simulink model "tutorial_switched_nets"  (R2020a)
settings: Solver=FixedStepAuto  StartTime=0.0  StopTime=options.T_train  FixedStep=options.dt  MaxStep=.2  RelTol=1e-3
model workspace (MAT data in the model file):
  PID_TRESH = 0.3
undefined symbols (not defined in the file or in its folder): DiscIntNeverNeededParam, options
libraries: neural x72, simulink x2
(part 2 of 3)

== system tutorial_switched_nets/NN/Layer 2/Delays 1 ==
  "p{2}" : Inport  PortDimensions=20
      mask Display: e = 0.06;c1 = [120 230 180]/255;c2 = ([120 230 180]+0)/(256+128);c3 = ([120 230 180]+128)/(256+128);patch([0 1 1 0],[0 0 1 1],c1);patch([0 1 1 1-e 1-e 0+e],[0 0 1 1-e 0+e 0+e],c2);patch([0 0 1 1-e 0+e 0+e],[0 1 1 1-e 1-e 0+e],c3);plot([0 1 1 0 0],[0 0 1 1 0]);
  mux : Mux  Inputs=1
      mask Display: e = 0.06;c1 = [120 150 230]/255;c2 = ([120 150 230]+0)/383;c3 = ([120 150 230]+128)/383;patch([0 1 1 0],[0 0 1 1],c1);patch([0 1 1 1-e 1-e 0+e],[0 0 1 1-e 0+e 0+e],c2);patch([0 0 1 1-e 0+e 0+e],[0 1 1 1-e 1-e 0+e],c3);plot([0 1 1 0 0],[0 0 1 1 0]);disp('Mux')
  "pd{2,1}" : Outport
      mask Display: e = 0.06;c1 = [120 230 180]/255;c2 = ([120 230 180]+0)/(256+128);c3 = ([120 230 180]+128)/(256+128);patch([0 1 1 0],[0 0 1 1],c1);patch([0 1 1 1-e 1-e 0+e],[0 0 1 1-e 0+e 0+e],c2);patch([0 0 1 1-e 0+e 0+e],[0 1 1 1-e 1-e 0+e],c3);plot([0 1 1 0 0],[0 0 1 1 0]);
  wires:
  "p{2}"/1 -> mux/1
  mux/1 -> "pd{2,1}"/1

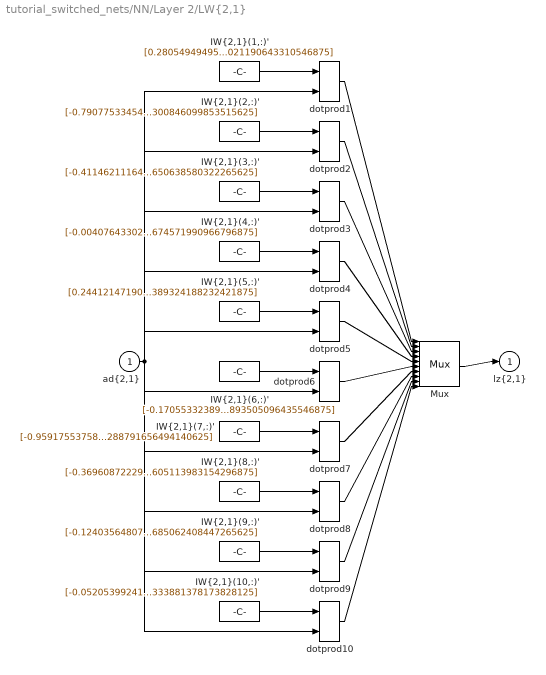
== system tutorial_switched_nets/NN/Layer 2/LW{2,1} ==
  "ad{2,1}" : Inport  PortDimensions=20
      mask Display: e = 0.06;c1 = [120 230 180]/255;c2 = ([120 230 180]+0)/(256+128);c3 = ([120 230 180]+128)/(256+128);patch([0 1 1 0],[0 0 1 1],c1);patch([0 1 1 1-e 1-e 0+e],[0 0 1 1-e 0+e 0+e],c2);patch([0 0 1 1-e 0+e 0+e],[0 1 1 1-e 1-e 0+e],c3);plot([0 1 1 0 0],[0 0 1 1 0]);
  "IW{2,1}(1,:)'" : Constant  Value=[0.280549494956085887498176134613458998501300811767578125;-0.459463207235249859738956956789479590952396392822265625;-0.7145226100256600876292623070185072720050811767578125;-0.66776447168319830183236263110302388668060302734375;0.28200698656808409481300259358249604701995849609375;0.281315192228172861188539854992995969951152801513671875;-0.1618202311625689671092942489849519915878772735595703125;-0.63712213282170504502488483922206796705722808837890625;0.64616452562049941921173967784852720797061920166015625;-0.236737456647389044039897498805657960474491119384765625;0.52016490423055483649505958965164609253406524658203125;-0.66477997520341325365933471402968280017375946044921875;0.2655032555560101759084545847144909203052520751953125;0.64607026299887115872166987173841334879398345947265625;-0.04869858942564757320337065493731643073260784149169921875;0.42144996396179801312342760866158641874790191650390625;-0.2978858712501490924040581376175396144390106201171875;-0.302468640537341071361510103088221512734889984130859375;-0.0760908416100260220904516472728573717176914215087890625;-0.37048121459967642277177901632967405021190643310546875]
      mask Display: e = 0.06;c1 = [120 150 230]/255;c2 = ([120 150 230]+0)/383;c3 = ([120 150 230]+128)/383;patch([0 1 1 0],[0 0 1 1],c1);patch([0 1 1 1-e 1-e 0+e],[0 0 1 1-e 0+e 0+e],c2);patch([0 0 1 1-e 0+e 0+e],[0 1 1 1-e 1-e 0+e],c3);plot([0 1 1 0 0],[0 0 1 1 0]);disp('weights');
  "IW{2,1}(10,:)'" : Constant  Value=[-0.05205399241633647255955708033070550300180912017822265625;0.5387685465762703795888910462963394820690155029296875;-0.75905182037552088036846953400527127087116241455078125;0.412938428245673561090001157936058007180690765380859375;-0.368082549618828525073155333302565850317478179931640625;0.11126545593356496066661520671914331614971160888671875;2.003689465912327438701368009787984192371368408203125;-1.3765062171366164722741132209193892776966094970703125;-0.400437914393512117694484686580835841596126556396484375;-0.460082361520731286663732362285372801125049591064453125;-0.335413367104632154092058726746472530066967010498046875;-0.2829915153567525987199360315571539103984832763671875;0.472274289772027844325208434383966960012912750244140625;-0.1443780989874181852616885635143262334167957305908203125;0.22917379984562569195105652397614903748035430908203125;-0.354072475071160130966063661617226898670196533203125;-0.0198754961378156506934811176279254141263663768768310546875;-0.385602437903931727358752823420218192040920257568359375;0.2184937935139707743115167204450699500739574432373046875;0.11170339781085758534828755728085525333881378173828125]
      mask Display: e = 0.06;c1 = [120 150 230]/255;c2 = ([120 150 230]+0)/383;c3 = ([120 150 230]+128)/383;patch([0 1 1 0],[0 0 1 1],c1);patch([0 1 1 1-e 1-e 0+e],[0 0 1 1-e 0+e 0+e],c2);patch([0 0 1 1-e 0+e 0+e],[0 1 1 1-e 1-e 0+e],c3);plot([0 1 1 0 0],[0 0 1 1 0]);disp('weights');
  "IW{2,1}(2,:)'" : Constant  Value=[-0.79077533454529491674378505194908939301967620849609375;-0.74867717022633140100396076377364806830883026123046875;0.65176919906250863068208900585887022316455841064453125;0.56218843471715640447428086190484464168548583984375;0.254249150001536194931617274050950072705745697021484375;-0.305788085839387713260606460607959888875484466552734375;0.1819051080462446290386679947914672084152698516845703125;-0.71683173127650035016955598621279932558536529541015625;0.0363478831189515128041733760255738161504268646240234375;0.483793083161081882703768997089355252683162689208984375;0.1366400352140867135997126524671330116689205169677734375;-0.00555997328650888709977717638821559376083314418792724609375;-0.5090116227204728449606818685424514114856719970703125;-0.1950975512537443667948622305630124174058437347412109375;0.377845845302065164172944378151441924273967742919921875;-0.09533470188304793424549643532373011112213134765625;1.0093380341353872520215873009874485433101654052734375;-0.11682982907864147836818347059306688606739044189453125;0.6836681441864487229764790754416026175022125244140625;-0.12217252125195900147591743234443129040300846099853515625]
      mask Display: e = 0.06;c1 = [120 150 230]/255;c2 = ([120 150 230]+0)/383;c3 = ([120 150 230]+128)/383;patch([0 1 1 0],[0 0 1 1],c1);patch([0 1 1 1-e 1-e 0+e],[0 0 1 1-e 0+e 0+e],c2);patch([0 0 1 1-e 0+e 0+e],[0 1 1 1-e 1-e 0+e],c3);plot([0 1 1 0 0],[0 0 1 1 0]);disp('weights');
  "IW{2,1}(3,:)'" : Constant  Value=[-0.411462111640641559073827693282510153949260711669921875;0.346422768199416974965743065695278346538543701171875;0.321500744716080311125239177272305823862552642822265625;-0.319829305919901496491064563088002614676952362060546875;-0.58753972953205868545722978524281643331050872802734375;-0.45520901850184625203610266908071935176849365234375;-0.057739648168344044620869937034512986429035663604736328125;0.26209508798584912891982412475044839084148406982421875;0.2373838621272965909714258714302559383213520050048828125;0.382322574360605849097538566638831980526447296142578125;-0.464968579933874470722088290131068788468837738037109375;-0.375021741146072062900174159949528984725475311279296875;-0.241437665265022527449900735518895089626312255859375;-0.0718540540957563755863901633347268216311931610107421875;0.249605496400429005543486482565640471875667572021484375;-0.467806927443950193445942886683042161166667938232421875;0.55601040814586821792175896916887722909450531005859375;0.1789510105579144028098426133510656654834747314453125;-0.54739428337578732719492791147786192595958709716796875;-0.1925896162076544959607105056420550681650638580322265625]
      mask Display: e = 0.06;c1 = [120 150 230]/255;c2 = ([120 150 230]+0)/383;c3 = ([120 150 230]+128)/383;patch([0 1 1 0],[0 0 1 1],c1);patch([0 1 1 1-e 1-e 0+e],[0 0 1 1-e 0+e 0+e],c2);patch([0 0 1 1-e 0+e 0+e],[0 1 1 1-e 1-e 0+e],c3);plot([0 1 1 0 0],[0 0 1 1 0]);disp('weights');
  "IW{2,1}(4,:)'" : Constant  Value=[-0.004076433029531396391720310390383019694127142429351806640625;0.1351551139496553199936812461601221002638339996337890625;0.1877537152214087401436160007506259717047214508056640625;0.67209099303780572842725860027712769806385040283203125;0.07648839395525099116301959156771772541105747222900390625;-0.2167608141488852890876870560532552190124988555908203125;1.1741853028082680499011303254519589245319366455078125;-0.74643004772053311857149537900113500654697418212890625;0.004784505717873065340495219999183973413892090320587158203125;0.438221873846528719997905909622204490005970001220703125;-0.15817284015984423017897597674163989722728729248046875;-0.1734443800270394631102277571699232794344425201416015625;0.460251097866992420204468317024293355643749237060546875;-0.66981204882548295298505536266020499169826507568359375;-0.66397302781903155821652262602583505213260650634765625;-0.432121736354837471250078806406236253678798675537109375;-0.439255382115188997005361670744605362415313720703125;0.441798550815553969783877619192935526371002197265625;-0.1843934156623856512879910951596684753894805908203125;-0.06502113910968147780788939371632295660674571990966796875]
      mask Display: e = 0.06;c1 = [120 150 230]/255;c2 = ([120 150 230]+0)/383;c3 = ([120 150 230]+128)/383;patch([0 1 1 0],[0 0 1 1],c1);patch([0 1 1 1-e 1-e 0+e],[0 0 1 1-e 0+e 0+e],c2);patch([0 0 1 1-e 0+e 0+e],[0 1 1 1-e 1-e 0+e],c3);plot([0 1 1 0 0],[0 0 1 1 0]);disp('weights');
  "IW{2,1}(5,:)'" : Constant  Value=[0.24412147190493860282600735445157624781131744384765625;-0.028459660312943800553053819157867110334336757659912109375;0.7242699730141033409580586521769873797893524169921875;-0.07029867854384859449101696782236103899776935577392578125;-0.20396990488081778725160120302462019026279449462890625;-0.3793777954263324314609917564666830003261566162109375;0.31381104904922685339130339343682862818241119384765625;-0.169479217191528752639584354255930520594120025634765625;-0.381243521182915323652906636198167689144611358642578125;0.993861801288782320540349246584810316562652587890625;0.1688437063823471639967266355597530491650104522705078125;0.055584824182623858435103869624072103761136531829833984375;0.233913992383819380194154291530139744281768798828125;-0.2774227486235549822168877653894014656543731689453125;0.044857182401254837300630384788746596314013004302978515625;-0.173384702362140930009815065204747952520847320556640625;0.019799159719305702009872760527287027798593044281005859375;0.577809908892843449024212532094679772853851318359375;0.1208540414982469390903219164101756177842617034912109375;-0.0215303846060126806427614809535953099839389324188232421875]
      mask Display: e = 0.06;c1 = [120 150 230]/255;c2 = ([120 150 230]+0)/383;c3 = ([120 150 230]+128)/383;patch([0 1 1 0],[0 0 1 1],c1);patch([0 1 1 1-e 1-e 0+e],[0 0 1 1-e 0+e 0+e],c2);patch([0 0 1 1-e 0+e 0+e],[0 1 1 1-e 1-e 0+e],c3);plot([0 1 1 0 0],[0 0 1 1 0]);disp('weights');
  "IW{2,1}(6,:)'" : Constant  Value=[-0.170553323894351571698990710501675494015216827392578125;0.315100169128914753269299353632959537208080291748046875;-0.0695263670126513577685045675025321543216705322265625;0.56233411969218638493117623511352576315402984619140625;1.09490589897904211369450422353111207485198974609375;0.51517503355886262728091651297290809452533721923828125;0.1585330202223078355228125246867421083152294158935546875;-0.306903270354190238489167086299858056008815765380859375;-0.06868717177946086216433485560628469102084636688232421875;0.5735024912398578589289854789967648684978485107421875;0.085519610363877174297186911644530482590198516845703125;0.3449989208232844273283035363419912755489349365234375;0.321257439517356913061263412600965239107608795166015625;0.6573053034924907223057743976823985576629638671875;-0.4424387215014797813950053750886581838130950927734375;-0.397036509305799756308630321655073203146457672119140625;-0.416827893457925091613702761605964042246341705322265625;-0.42478000989293918099320990222622640430927276611328125;0.41805630426794204712592772921198047697544097900390625;-0.0152415151666972052690862682311490061692893505096435546875]
      mask Display: e = 0.06;c1 = [120 150 230]/255;c2 = ([120 150 230]+0)/383;c3 = ([120 150 230]+128)/383;patch([0 1 1 0],[0 0 1 1],c1);patch([0 1 1 1-e 1-e 0+e],[0 0 1 1-e 0+e 0+e],c2);patch([0 0 1 1-e 0+e 0+e],[0 1 1 1-e 1-e 0+e],c3);plot([0 1 1 0 0],[0 0 1 1 0]);disp('weights');
  "IW{2,1}(7,:)'" : Constant  Value=[-0.9591755375881791945147369915503077208995819091796875;0.478966355111692998480776850556139834225177764892578125;0.327451054909865646447286735565285198390483856201171875;0.472977571176947331199613699936890043318271636962890625;-0.280248343611868400149234048512880690395832061767578125;0.299821012346937421089165809462429024279117584228515625;-0.539468324559729150990960988565348088741302490234375;-0.70262854824193488045835920274839736521244049072265625;0.585742309266132910039459602558054029941558837890625;-0.349443377561848789181198071673861704766750335693359375;-1.221770236197789127885471316403709352016448974609375;0.1224367331808378922541891142827807925641536712646484375;-1.030639550776817348065605983720161020755767822265625;-0.1693463759913551580638113591703586280345916748046875;0.10265330909329183073364077927180915139615535736083984375;0.53961251266413678973066225807997398078441619873046875;-0.57714196282421481587476819186122156679630279541015625;0.7088290553452194497907612458220683038234710693359375;-0.12987398737049338226512418259517289698123931884765625;0.379163849590473278627911213334300555288791656494140625]
      mask Display: e = 0.06;c1 = [120 150 230]/255;c2 = ([120 150 230]+0)/383;c3 = ([120 150 230]+128)/383;patch([0 1 1 0],[0 0 1 1],c1);patch([0 1 1 1-e 1-e 0+e],[0 0 1 1-e 0+e 0+e],c2);patch([0 0 1 1-e 0+e 0+e],[0 1 1 1-e 1-e 0+e],c3);plot([0 1 1 0 0],[0 0 1 1 0]);disp('weights');
  "IW{2,1}(8,:)'" : Constant  Value=[-0.369608722297072145313023838752997107803821563720703125;-0.42838684570988672106750527746044099330902099609375;0.01479004215599865994235084798447132925502955913543701171875;0.391470456224183360749435678371810354292392730712890625;0.05716198700565870705059268175318720750510692596435546875;0.455286775660560250056363429393968544900417327880859375;-0.40994265952623709647895111629622988402843475341796875;0.004042807168400087969306611057618283666670322418212890625;-0.1858221076821540418411160544565063901245594024658203125;0.024868606478489797828590468498077825643122196197509765625;0.06550058497320099260008419150835834443569183349609375;-0.05485708254809618100722445888095535337924957275390625;-0.04984332589573468863530791850280365906655788421630859375;-0.264291657102464883077885815509944222867488861083984375;-0.51002433505330568852542683089268393814563751220703125;-0.41083929437252908467570478023844771087169647216796875;0.07118183415549168835401161459230934269726276397705078125;-0.345966143720376095860302712026168592274188995361328125;-0.004967097276482514145445890108021558262407779693603515625;0.10225962854229846132891879051385330967605113983154296875]
      mask Display: e = 0.06;c1 = [120 150 230]/255;c2 = ([120 150 230]+0)/383;c3 = ([120 150 230]+128)/383;patch([0 1 1 0],[0 0 1 1],c1);patch([0 1 1 1-e 1-e 0+e],[0 0 1 1-e 0+e 0+e],c2);patch([0 0 1 1-e 0+e 0+e],[0 1 1 1-e 1-e 0+e],c3);plot([0 1 1 0 0],[0 0 1 1 0]);disp('weights');
  "IW{2,1}(9,:)'" : Constant  Value=[-0.12403564807650326040633359525600099004805088043212890625;-0.3813918034744816498715636043925769627094268798828125;-0.5403292331634332867906778119504451751708984375;-0.399293688240054234217524253836018033325672149658203125;-0.2594835850826997525331307770102284848690032958984375;0.1750587736692832407925379811786115169525146484375;-0.419700000664224359692155985612771473824977874755859375;-0.1189769142623696429605928415185189805924892425537109375;0.316449424162375370084276937632239423692226409912109375;0.57027604509409968169819649119745008647441864013671875;0.4994740777990991364987394263152964413166046142578125;-0.36276934641806579673328769786166958510875701904296875;-0.447938247529432842508612111487309448421001434326171875;-0.165673007270111749544838630754384212195873260498046875;0.84050803965784715021669626366929151117801666259765625;0.141349907709793887189420047434396110475063323974609375;0.2151272861102743461092501320308656431734561920166015625;0.080626987507818992373387345651281066238880157470703125;-1.5993299783241570199976422372856177389621734619140625;0.77587111661611152246820211075828410685062408447265625]
      mask Display: e = 0.06;c1 = [120 150 230]/255;c2 = ([120 150 230]+0)/383;c3 = ([120 150 230]+128)/383;patch([0 1 1 0],[0 0 1 1],c1);patch([0 1 1 1-e 1-e 0+e],[0 0 1 1-e 0+e 0+e],c2);patch([0 0 1 1-e 0+e 0+e],[0 1 1 1-e 1-e 0+e],c3);plot([0 1 1 0 0],[0 0 1 1 0]);disp('weights');
  Mux : Mux  Inputs=10
      mask Display: e = 0.06;c1 = [120 150 230]/255;c2 = ([120 150 230]+0)/383;c3 = ([120 150 230]+128)/383;patch([0 1 1 0],[0 0 1 1],c1);patch([0 1 1 1-e 1-e 0+e],[0 0 1 1-e 0+e 0+e],c2);patch([0 0 1 1-e 0+e 0+e],[0 1 1 1-e 1-e 0+e],c3);plot([0 1 1 0 0],[0 0 1 1 0]);disp('Mux');
  dotprod{1..10} (10 alike) : neural/Weight Functions/dotprod
  "lz{2,1}" : Outport
      mask Display: e = 0.06;c1 = [120 230 180]/255;c2 = ([120 230 180]+0)/(256+128);c3 = ([120 230 180]+128)/(256+128);patch([0 1 1 0],[0 0 1 1],c1);patch([0 1 1 1-e 1-e 0+e],[0 0 1 1-e 0+e 0+e],c2);patch([0 0 1 1-e 0+e 0+e],[0 1 1 1-e 1-e 0+e],c3);plot([0 1 1 0 0],[0 0 1 1 0]);
  wires:
  "IW{2,1}(1,:)'"/1 -> dotprod1/1
  "ad{2,1}"/1 -> dotprod1/2, dotprod2/2, dotprod3/2, dotprod4/2, dotprod5/2, dotprod6/2, dotprod7/2, dotprod8/2, dotprod9/2, dotprod10/2
  dotprod1/1 -> Mux/1
  "IW{2,1}(2,:)'"/1 -> dotprod2/1
  dotprod2/1 -> Mux/2
  "IW{2,1}(3,:)'"/1 -> dotprod3/1
  dotprod3/1 -> Mux/3
  "IW{2,1}(4,:)'"/1 -> dotprod4/1
  dotprod4/1 -> Mux/4
  "IW{2,1}(5,:)'"/1 -> dotprod5/1
  dotprod5/1 -> Mux/5
  "IW{2,1}(6,:)'"/1 -> dotprod6/1
  dotprod6/1 -> Mux/6
  "IW{2,1}(7,:)'"/1 -> dotprod7/1
  dotprod7/1 -> Mux/7
  "IW{2,1}(8,:)'"/1 -> dotprod8/1
  dotprod8/1 -> Mux/8
  "IW{2,1}(9,:)'"/1 -> dotprod9/1
  dotprod9/1 -> Mux/9
  "IW{2,1}(10,:)'"/1 -> dotprod10/1
  dotprod10/1 -> Mux/10
  Mux/1 -> "lz{2,1}"/1

== system tutorial_switched_nets/NN/Layer 3/Delays 1 ==
  "p{3}" : Inport  PortDimensions=10
      mask Display: e = 0.06;c1 = [120 230 180]/255;c2 = ([120 230 180]+0)/(256+128);c3 = ([120 230 180]+128)/(256+128);patch([0 1 1 0],[0 0 1 1],c1);patch([0 1 1 1-e 1-e 0+e],[0 0 1 1-e 0+e 0+e],c2);patch([0 0 1 1-e 0+e 0+e],[0 1 1 1-e 1-e 0+e],c3);plot([0 1 1 0 0],[0 0 1 1 0]);
  mux : Mux  Inputs=1
      mask Display: e = 0.06;c1 = [120 150 230]/255;c2 = ([120 150 230]+0)/383;c3 = ([120 150 230]+128)/383;patch([0 1 1 0],[0 0 1 1],c1);patch([0 1 1 1-e 1-e 0+e],[0 0 1 1-e 0+e 0+e],c2);patch([0 0 1 1-e 0+e 0+e],[0 1 1 1-e 1-e 0+e],c3);plot([0 1 1 0 0],[0 0 1 1 0]);disp('Mux')
  "pd{3,2}" : Outport
      mask Display: e = 0.06;c1 = [120 230 180]/255;c2 = ([120 230 180]+0)/(256+128);c3 = ([120 230 180]+128)/(256+128);patch([0 1 1 0],[0 0 1 1],c1);patch([0 1 1 1-e 1-e 0+e],[0 0 1 1-e 0+e 0+e],c2);patch([0 0 1 1-e 0+e 0+e],[0 1 1 1-e 1-e 0+e],c3);plot([0 1 1 0 0],[0 0 1 1 0]);
  wires:
  "p{3}"/1 -> mux/1
  mux/1 -> "pd{3,2}"/1

== system tutorial_switched_nets/NN/Layer 3/LW{3,2} ==
  "ad{3,2}" : Inport  PortDimensions=10
      mask Display: e = 0.06;c1 = [120 230 180]/255;c2 = ([120 230 180]+0)/(256+128);c3 = ([120 230 180]+128)/(256+128);patch([0 1 1 0],[0 0 1 1],c1);patch([0 1 1 1-e 1-e 0+e],[0 0 1 1-e 0+e 0+e],c2);patch([0 0 1 1-e 0+e 0+e],[0 1 1 1-e 1-e 0+e],c3);plot([0 1 1 0 0],[0 0 1 1 0]);
  "IW{3,2}(1,:)'" : Constant  Value=[-0.322573760839003187417262097369530238211154937744140625;1.3381484741628077994590739763225428760051727294921875;-0.380101450462710044320147062535397708415985107421875;-1.5890428350951062430596039121155627071857452392578125;-0.55620301261056492858614319629850797355175018310546875;0.71401750856864609762197915188153274357318878173828125;-0.604571533080045409036529235891066491603851318359375;-0.86505758880961736156933739039232023060321807861328125;-0.56217279130365349626430315765901468694210052490234375;1.554871021080632242927777042496018111705780029296875]
      mask Display: e = 0.06;c1 = [120 150 230]/255;c2 = ([120 150 230]+0)/383;c3 = ([120 150 230]+128)/383;patch([0 1 1 0],[0 0 1 1],c1);patch([0 1 1 1-e 1-e 0+e],[0 0 1 1-e 0+e 0+e],c2);patch([0 0 1 1-e 0+e 0+e],[0 1 1 1-e 1-e 0+e],c3);plot([0 1 1 0 0],[0 0 1 1 0]);disp('weights');
  Mux : Mux  Inputs=1
      mask Display: e = 0.06;c1 = [120 150 230]/255;c2 = ([120 150 230]+0)/383;c3 = ([120 150 230]+128)/383;patch([0 1 1 0],[0 0 1 1],c1);patch([0 1 1 1-e 1-e 0+e],[0 0 1 1-e 0+e 0+e],c2);patch([0 0 1 1-e 0+e 0+e],[0 1 1 1-e 1-e 0+e],c3);plot([0 1 1 0 0],[0 0 1 1 0]);disp('Mux');
  dotprod1 : neural/Weight Functions/dotprod
  "lz{3,2}" : Outport
      mask Display: e = 0.06;c1 = [120 230 180]/255;c2 = ([120 230 180]+0)/(256+128);c3 = ([120 230 180]+128)/(256+128);patch([0 1 1 0],[0 0 1 1],c1);patch([0 1 1 1-e 1-e 0+e],[0 0 1 1-e 0+e 0+e],c2);patch([0 0 1 1-e 0+e 0+e],[0 1 1 1-e 1-e 0+e],c3);plot([0 1 1 0 0],[0 0 1 1 0]);
  wires:
  "IW{3,2}(1,:)'"/1 -> dotprod1/1
  "ad{3,2}"/1 -> dotprod1/2
  dotprod1/1 -> Mux/1
  Mux/1 -> "lz{3,2}"/1

== system tutorial_switched_nets/NN_cex_1/Layer 1/Delays 1 ==
  "p{1}" : Inport  PortDimensions=6
      mask Display: e = 0.06;c1 = [120 230 180]/255;c2 = ([120 230 180]+0)/(256+128);c3 = ([120 230 180]+128)/(256+128);patch([0 1 1 0],[0 0 1 1],c1);patch([0 1 1 1-e 1-e 0+e],[0 0 1 1-e 0+e 0+e],c2);patch([0 0 1 1-e 0+e 0+e],[0 1 1 1-e 1-e 0+e],c3);plot([0 1 1 0 0],[0 0 1 1 0]);
  mux : Mux  Inputs=1
      mask Display: e = 0.06;c1 = [120 150 230]/255;c2 = ([120 150 230]+0)/383;c3 = ([120 150 230]+128)/383;patch([0 1 1 0],[0 0 1 1],c1);patch([0 1 1 1-e 1-e 0+e],[0 0 1 1-e 0+e 0+e],c2);patch([0 0 1 1-e 0+e 0+e],[0 1 1 1-e 1-e 0+e],c3);plot([0 1 1 0 0],[0 0 1 1 0]);disp('Mux')
  "pd{1,1}" : Outport
      mask Display: e = 0.06;c1 = [120 230 180]/255;c2 = ([120 230 180]+0)/(256+128);c3 = ([120 230 180]+128)/(256+128);patch([0 1 1 0],[0 0 1 1],c1);patch([0 1 1 1-e 1-e 0+e],[0 0 1 1-e 0+e 0+e],c2);patch([0 0 1 1-e 0+e 0+e],[0 1 1 1-e 1-e 0+e],c3);plot([0 1 1 0 0],[0 0 1 1 0]);
  wires:
  "p{1}"/1 -> mux/1
  mux/1 -> "pd{1,1}"/1

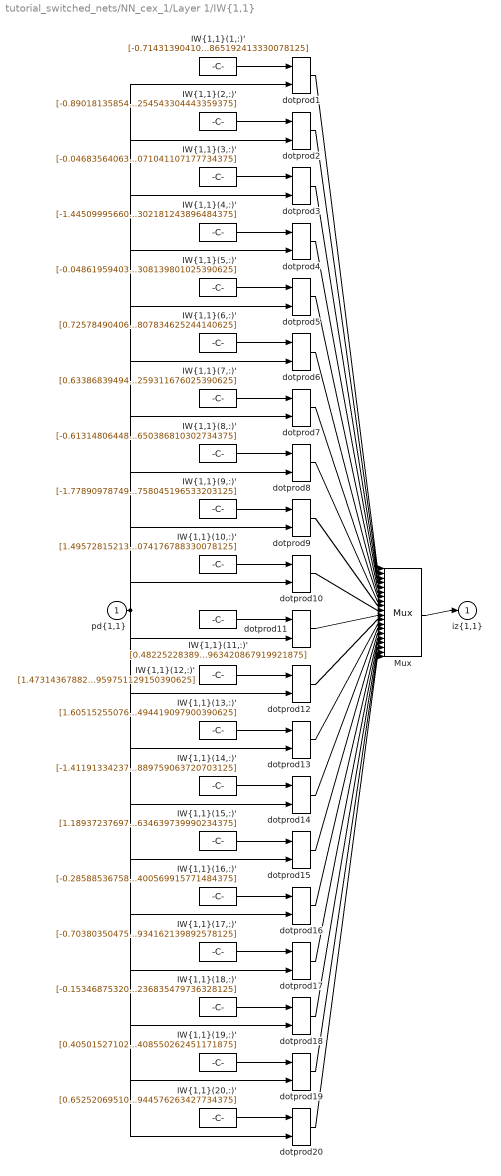
== system tutorial_switched_nets/NN_cex_1/Layer 1/IW{1,1} ==
  "pd{1,1}" : Inport  PortDimensions=6
      mask Display: e = 0.06;c1 = [120 230 180]/255;c2 = ([120 230 180]+0)/(256+128);c3 = ([120 230 180]+128)/(256+128);patch([0 1 1 0],[0 0 1 1],c1);patch([0 1 1 1-e 1-e 0+e],[0 0 1 1-e 0+e 0+e],c2);patch([0 0 1 1-e 0+e 0+e],[0 1 1 1-e 1-e 0+e],c3);plot([0 1 1 0 0],[0 0 1 1 0]);
  "IW{1,1}(1,:)'" : Constant  Value=[-0.7143139041002670719393563558696769177913665771484375;-1.1942528110373960004153559566475450992584228515625;1.4196286055412679072418313808157108724117279052734375;0.6987335842010169439930677981465123593807220458984375;0.481917919156309049188990911716246046125888824462890625;1.241612815635754873966334344004280865192413330078125]
      mask Display: e = 0.06;c1 = [120 150 230]/255;c2 = ([120 150 230]+0)/383;c3 = ([120 150 230]+128)/383;patch([0 1 1 0],[0 0 1 1],c1);patch([0 1 1 1-e 1-e 0+e],[0 0 1 1-e 0+e 0+e],c2);patch([0 0 1 1-e 0+e 0+e],[0 1 1 1-e 1-e 0+e],c3);plot([0 1 1 0 0],[0 0 1 1 0]);disp('Weights');
  "IW{1,1}(10,:)'" : Constant  Value=[1.4957281521381233790890519230742938816547393798828125;-0.4124038460344738865614999667741358280181884765625;-0.351826835250488023643100632398272864520549774169921875;-1.391849838246075332648388211964629590511322021484375;0.6728593524781529833234117177198641002178192138671875;-0.07799088896193062669937035025213845074176788330078125]
      mask Display: e = 0.06;c1 = [120 150 230]/255;c2 = ([120 150 230]+0)/383;c3 = ([120 150 230]+128)/383;patch([0 1 1 0],[0 0 1 1],c1);patch([0 1 1 1-e 1-e 0+e],[0 0 1 1-e 0+e 0+e],c2);patch([0 0 1 1-e 0+e 0+e],[0 1 1 1-e 1-e 0+e],c3);plot([0 1 1 0 0],[0 0 1 1 0]);disp('Weights');
  "IW{1,1}(11,:)'" : Constant  Value=[0.482252283894366140515330698690377175807952880859375;-0.8692007105892205487407409236766397953033447265625;1.8789470571170683310668891863315366208553314208984375;-0.5684388765228376438898294509272091090679168701171875;-0.9088965431518232218621733409236185252666473388671875;-0.59981150125534987704867262436891905963420867919921875]
      mask Display: e = 0.06;c1 = [120 150 230]/255;c2 = ([120 150 230]+0)/383;c3 = ([120 150 230]+128)/383;patch([0 1 1 0],[0 0 1 1],c1);patch([0 1 1 1-e 1-e 0+e],[0 0 1 1-e 0+e 0+e],c2);patch([0 0 1 1-e 0+e 0+e],[0 1 1 1-e 1-e 0+e],c3);plot([0 1 1 0 0],[0 0 1 1 0]);disp('Weights');
  "IW{1,1}(12,:)'" : Constant  Value=[1.473143678827943059417293625301681458950042724609375;-1.5301503648807097679451771909953095018863677978515625;-0.63431129302834221572737760652671568095684051513671875;0.126823507792890366463467444191337563097476959228515625;-0.482306692662358649226206352977897040545940399169921875;1.2564718652289850187031561290496028959751129150390625]
      mask Display: e = 0.06;c1 = [120 150 230]/255;c2 = ([120 150 230]+0)/383;c3 = ([120 150 230]+128)/383;patch([0 1 1 0],[0 0 1 1],c1);patch([0 1 1 1-e 1-e 0+e],[0 0 1 1-e 0+e 0+e],c2);patch([0 0 1 1-e 0+e 0+e],[0 1 1 1-e 1-e 0+e],c3);plot([0 1 1 0 0],[0 0 1 1 0]);disp('Weights');
  "IW{1,1}(13,:)'" : Constant  Value=[1.6051525507621864363727581803686916828155517578125;0.98898767359491868145227044806233607232570648193359375;3.108475425991156892990829874179325997829437255859375;-2.472151701812612234476773664937354624271392822265625;-1.653892040361615745069912009057588875293731689453125;-2.35596887353649098173491438501514494419097900390625]
      mask Display: e = 0.06;c1 = [120 150 230]/255;c2 = ([120 150 230]+0)/383;c3 = ([120 150 230]+128)/383;patch([0 1 1 0],[0 0 1 1],c1);patch([0 1 1 1-e 1-e 0+e],[0 0 1 1-e 0+e 0+e],c2);patch([0 0 1 1-e 0+e 0+e],[0 1 1 1-e 1-e 0+e],c3);plot([0 1 1 0 0],[0 0 1 1 0]);disp('Weights');
  "IW{1,1}(14,:)'" : Constant  Value=[-1.411913342371418966791907223523594439029693603515625;-0.09908892325603159412228393421173677779734134674072265625;0.38794016675093023760467758620507083833217620849609375;0.214080978566828339371141964875278063118457794189453125;1.426095767275657788530907055246643722057342529296875;2.243067793217360605950716490042395889759063720703125]
      mask Display: e = 0.06;c1 = [120 150 230]/255;c2 = ([120 150 230]+0)/383;c3 = ([120 150 230]+128)/383;patch([0 1 1 0],[0 0 1 1],c1);patch([0 1 1 1-e 1-e 0+e],[0 0 1 1-e 0+e 0+e],c2);patch([0 0 1 1-e 0+e 0+e],[0 1 1 1-e 1-e 0+e],c3);plot([0 1 1 0 0],[0 0 1 1 0]);disp('Weights');
  "IW{1,1}(15,:)'" : Constant  Value=[1.189372376979445089517639644327573478221893310546875;-0.63676217811669444390787475640536285936832427978515625;-1.0607441335999379106169726583175361156463623046875;1.107813751652075406894937259494327008724212646484375;-0.77649458456781872417451495493878610432147979736328125;-0.586501597742093760956549886032007634639739990234375]
      mask Display: e = 0.06;c1 = [120 150 230]/255;c2 = ([120 150 230]+0)/383;c3 = ([120 150 230]+128)/383;patch([0 1 1 0],[0 0 1 1],c1);patch([0 1 1 1-e 1-e 0+e],[0 0 1 1-e 0+e 0+e],c2);patch([0 0 1 1-e 0+e 0+e],[0 1 1 1-e 1-e 0+e],c3);plot([0 1 1 0 0],[0 0 1 1 0]);disp('Weights');
  "IW{1,1}(16,:)'" : Constant  Value=[-0.285885367587746908046852922780090011656284332275390625;1.6224546591903157288783177136792801320552825927734375;-0.301397424443253958425970040480024181306362152099609375;0.9006938286797281367768164273002184927463531494140625;0.140546397019933821948001195778488181531429290771484375;1.5223707118062195231544819762348197400569915771484375]
      mask Display: e = 0.06;c1 = [120 150 230]/255;c2 = ([120 150 230]+0)/383;c3 = ([120 150 230]+128)/383;patch([0 1 1 0],[0 0 1 1],c1);patch([0 1 1 1-e 1-e 0+e],[0 0 1 1-e 0+e 0+e],c2);patch([0 0 1 1-e 0+e 0+e],[0 1 1 1-e 1-e 0+e],c3);plot([0 1 1 0 0],[0 0 1 1 0]);disp('Weights');
  "IW{1,1}(17,:)'" : Constant  Value=[-0.7038035047596438165129484332283027470111846923828125;-0.134545716086009570222614684098516590893268585205078125;0.6188616409972365062230892363004386425018310546875;-0.313747198053605236278684742501354776322841644287109375;1.3721403750456395709278467620606534183025360107421875;1.50954987246020255753364835982210934162139892578125]
      mask Display: e = 0.06;c1 = [120 150 230]/255;c2 = ([120 150 230]+0)/383;c3 = ([120 150 230]+128)/383;patch([0 1 1 0],[0 0 1 1],c1);patch([0 1 1 1-e 1-e 0+e],[0 0 1 1-e 0+e 0+e],c2);patch([0 0 1 1-e 0+e 0+e],[0 1 1 1-e 1-e 0+e],c3);plot([0 1 1 0 0],[0 0 1 1 0]);disp('Weights');
  "IW{1,1}(18,:)'" : Constant  Value=[-0.15346875320228392514110282718320377171039581298828125;-1.3856719607525020965255180271924473345279693603515625;1.6123731664722369405495783212245441973209381103515625;0.9810297090513941942191422640462405979633331298828125;0.418556892039820105377856407358194701373577117919921875;-1.0203540989074213474196994866360910236835479736328125]
      mask Display: e = 0.06;c1 = [120 150 230]/255;c2 = ([120 150 230]+0)/383;c3 = ([120 150 230]+128)/383;patch([0 1 1 0],[0 0 1 1],c1);patch([0 1 1 1-e 1-e 0+e],[0 0 1 1-e 0+e 0+e],c2);patch([0 0 1 1-e 0+e 0+e],[0 1 1 1-e 1-e 0+e],c3);plot([0 1 1 0 0],[0 0 1 1 0]);disp('Weights');
  "IW{1,1}(19,:)'" : Constant  Value=[0.40501527102416845504961884216754697263240814208984375;-1.1709579271866992211670321921701543033123016357421875;1.0390873452748063954231838579289615154266357421875;-0.9243501635854893816457433786126784980297088623046875;0.5186913221198772294684431471978314220905303955078125;-0.82731422783971353407395099566201679408550262451171875]
      mask Display: e = 0.06;c1 = [120 150 230]/255;c2 = ([120 150 230]+0)/383;c3 = ([120 150 230]+128)/383;patch([0 1 1 0],[0 0 1 1],c1);patch([0 1 1 1-e 1-e 0+e],[0 0 1 1-e 0+e 0+e],c2);patch([0 0 1 1-e 0+e 0+e],[0 1 1 1-e 1-e 0+e],c3);plot([0 1 1 0 0],[0 0 1 1 0]);disp('Weights');
  "IW{1,1}(2,:)'" : Constant  Value=[-0.89018135854567204123810597593546845018863677978515625;0.01533281723726308276578578215776360593736171722412109375;-1.864709008135601475686371486517600715160369873046875;-0.327973807444661480392511521131382323801517486572265625;-0.68741673613350362526119852191186510026454925537109375;-0.80715739731796387612661192179075442254543304443359375]
      mask Display: e = 0.06;c1 = [120 150 230]/255;c2 = ([120 150 230]+0)/383;c3 = ([120 150 230]+128)/383;patch([0 1 1 0],[0 0 1 1],c1);patch([0 1 1 1-e 1-e 0+e],[0 0 1 1-e 0+e 0+e],c2);patch([0 0 1 1-e 0+e 0+e],[0 1 1 1-e 1-e 0+e],c3);plot([0 1 1 0 0],[0 0 1 1 0]);disp('Weights');
  "IW{1,1}(20,:)'" : Constant  Value=[0.652520695109815473955450215726159512996673583984375;-0.5276878883598417058209406604873947799205780029296875;-0.219952293544739607700222450148430652916431427001953125;-0.94955447445423890595606053466326557099819183349609375;1.498409794110231008090750037808902561664581298828125;-0.6643653980759489652285765259875915944576263427734375]
      mask Display: e = 0.06;c1 = [120 150 230]/255;c2 = ([120 150 230]+0)/383;c3 = ([120 150 230]+128)/383;patch([0 1 1 0],[0 0 1 1],c1);patch([0 1 1 1-e 1-e 0+e],[0 0 1 1-e 0+e 0+e],c2);patch([0 0 1 1-e 0+e 0+e],[0 1 1 1-e 1-e 0+e],c3);plot([0 1 1 0 0],[0 0 1 1 0]);disp('Weights');
  "IW{1,1}(3,:)'" : Constant  Value=[-0.04683564063780364106204245899789384566247463226318359375;0.235368234207319615425291203791857697069644927978515625;0.34539956295796747642867785543785430490970611572265625;-1.1092919282513331591388805463793687522411346435546875;-0.95498722069700614500931123984628356993198394775390625;-0.65873863273703869847253145053400658071041107177734375]
      mask Display: e = 0.06;c1 = [120 150 230]/255;c2 = ([120 150 230]+0)/383;c3 = ([120 150 230]+128)/383;patch([0 1 1 0],[0 0 1 1],c1);patch([0 1 1 1-e 1-e 0+e],[0 0 1 1-e 0+e 0+e],c2);patch([0 0 1 1-e 0+e 0+e],[0 1 1 1-e 1-e 0+e],c3);plot([0 1 1 0 0],[0 0 1 1 0]);disp('Weights');
  "IW{1,1}(4,:)'" : Constant  Value=[-1.4450999566026616616198907649959437549114227294921875;1.4870643104817660162808579116244800388813018798828125;1.1697469559922824000608443384408019483089447021484375;-0.76372206543721732341367669505416415631771087646484375;0.0767838415232345583572026725960313342511653900146484375;-0.7949392016602290222948568043648265302181243896484375]
      mask Display: e = 0.06;c1 = [120 150 230]/255;c2 = ([120 150 230]+0)/383;c3 = ([120 150 230]+128)/383;patch([0 1 1 0],[0 0 1 1],c1);patch([0 1 1 1-e 1-e 0+e],[0 0 1 1-e 0+e 0+e],c2);patch([0 0 1 1-e 0+e 0+e],[0 1 1 1-e 1-e 0+e],c3);plot([0 1 1 0 0],[0 0 1 1 0]);disp('Weights');
  "IW{1,1}(5,:)'" : Constant  Value=[-0.0486195940395940662259732789607369340956211090087890625;-0.8195775409645733589059091173112392425537109375;-2.050021123198646488816621058504097163677215576171875;-0.045003064607668639973692137346006347797811031341552734375;-0.424666111229862253129141436147619970142841339111328125;-0.34850998634873031623016004232340492308139801025390625]
      mask Display: e = 0.06;c1 = [120 150 230]/255;c2 = ([120 150 230]+0)/383;c3 = ([120 150 230]+128)/383;patch([0 1 1 0],[0 0 1 1],c1);patch([0 1 1 1-e 1-e 0+e],[0 0 1 1-e 0+e 0+e],c2);patch([0 0 1 1-e 0+e 0+e],[0 1 1 1-e 1-e 0+e],c3);plot([0 1 1 0 0],[0 0 1 1 0]);disp('Weights');
  "IW{1,1}(6,:)'" : Constant  Value=[0.725784904069509906321400194428861141204833984375;-1.0642883254580091101360039829160086810588836669921875;1.0350943246672474895575533082592301070690155029296875;0.86389220677928990621552429729490540921688079833984375;-1.119068236744578115349213476292788982391357421875;-0.70058975029126546729685287573374807834625244140625]
      mask Display: e = 0.06;c1 = [120 150 230]/255;c2 = ([120 150 230]+0)/383;c3 = ([120 150 230]+128)/383;patch([0 1 1 0],[0 0 1 1],c1);patch([0 1 1 1-e 1-e 0+e],[0 0 1 1-e 0+e 0+e],c2);patch([0 0 1 1-e 0+e 0+e],[0 1 1 1-e 1-e 0+e],c3);plot([0 1 1 0 0],[0 0 1 1 0]);disp('Weights');
  "IW{1,1}(7,:)'" : Constant  Value=[0.63386839494892743829268511035479605197906494140625;-1.4396116977867248198919014612329192459583282470703125;-0.2411510510841359533618089017181773670017719268798828125;-0.59745680626877695207355145612382330000400543212890625;-1.38223838464698456363066725316457450389862060546875;-0.94315921171589389704337236253195442259311676025390625]
      mask Display: e = 0.06;c1 = [120 150 230]/255;c2 = ([120 150 230]+0)/383;c3 = ([120 150 230]+128)/383;patch([0 1 1 0],[0 0 1 1],c1);patch([0 1 1 1-e 1-e 0+e],[0 0 1 1-e 0+e 0+e],c2);patch([0 0 1 1-e 0+e 0+e],[0 1 1 1-e 1-e 0+e],c3);plot([0 1 1 0 0],[0 0 1 1 0]);disp('Weights');
  "IW{1,1}(8,:)'" : Constant  Value=[-0.61314806448595604582152418515761382877826690673828125;0.97330128297518825331025027480791322886943817138671875;1.22590446270022379593456207658164203166961669921875;-1.3697902995010216020688176286057569086551666259765625;-0.278979247034279509431797805518726818263530731201171875;-1.3025317160996416898655070326640270650386810302734375]
      mask Display: e = 0.06;c1 = [120 150 230]/255;c2 = ([120 150 230]+0)/383;c3 = ([120 150 230]+128)/383;patch([0 1 1 0],[0 0 1 1],c1);patch([0 1 1 1-e 1-e 0+e],[0 0 1 1-e 0+e 0+e],c2);patch([0 0 1 1-e 0+e 0+e],[0 1 1 1-e 1-e 0+e],c3);plot([0 1 1 0 0],[0 0 1 1 0]);disp('Weights');
  "IW{1,1}(9,:)'" : Constant  Value=[-1.77890978749349670806623180396854877471923828125;-1.9353132505466172919028622345649637281894683837890625;-1.7707139496077537454965522556449286639690399169921875;-0.31769325805262160766773149589425884187221527099609375;-0.5695700461881301190913973186980001628398895263671875;0.69769734755491452649067696256679482758045196533203125]
      mask Display: e = 0.06;c1 = [120 150 230]/255;c2 = ([120 150 230]+0)/383;c3 = ([120 150 230]+128)/383;patch([0 1 1 0],[0 0 1 1],c1);patch([0 1 1 1-e 1-e 0+e],[0 0 1 1-e 0+e 0+e],c2);patch([0 0 1 1-e 0+e 0+e],[0 1 1 1-e 1-e 0+e],c3);plot([0 1 1 0 0],[0 0 1 1 0]);disp('Weights');
  Mux : Mux  Inputs=20
      mask Display: e = 0.06;c1 = [120 150 230]/255;c2 = ([120 150 230]+0)/383;c3 = ([120 150 230]+128)/383;patch([0 1 1 0],[0 0 1 1],c1);patch([0 1 1 1-e 1-e 0+e],[0 0 1 1-e 0+e 0+e],c2);patch([0 0 1 1-e 0+e 0+e],[0 1 1 1-e 1-e 0+e],c3);plot([0 1 1 0 0],[0 0 1 1 0]);disp('Mux');
  dotprod{1..20} (20 alike) : neural/Weight Functions/dotprod
  "iz{1,1}" : Outport
      mask Display: e = 0.06;c1 = [120 230 180]/255;c2 = ([120 230 180]+0)/(256+128);c3 = ([120 230 180]+128)/(256+128);patch([0 1 1 0],[0 0 1 1],c1);patch([0 1 1 1-e 1-e 0+e],[0 0 1 1-e 0+e 0+e],c2);patch([0 0 1 1-e 0+e 0+e],[0 1 1 1-e 1-e 0+e],c3);plot([0 1 1 0 0],[0 0 1 1 0]);
  wires:
  "IW{1,1}(1,:)'"/1 -> dotprod1/1
  "pd{1,1}"/1 -> dotprod1/2, dotprod2/2, dotprod3/2, dotprod4/2, dotprod5/2, dotprod6/2, dotprod7/2, dotprod8/2, dotprod9/2, dotprod10/2, dotprod11/2, dotprod12/2, dotprod13/2, dotprod14/2, dotprod15/2, dotprod16/2, dotprod17/2, dotprod18/2, dotprod19/2, dotprod20/2
  dotprod1/1 -> Mux/1
  "IW{1,1}(2,:)'"/1 -> dotprod2/1
  dotprod2/1 -> Mux/2
  "IW{1,1}(3,:)'"/1 -> dotprod3/1
  dotprod3/1 -> Mux/3
  "IW{1,1}(4,:)'"/1 -> dotprod4/1
  dotprod4/1 -> Mux/4
  "IW{1,1}(5,:)'"/1 -> dotprod5/1
  dotprod5/1 -> Mux/5
  "IW{1,1}(6,:)'"/1 -> dotprod6/1
  dotprod6/1 -> Mux/6
  "IW{1,1}(7,:)'"/1 -> dotprod7/1
  dotprod7/1 -> Mux/7
  "IW{1,1}(8,:)'"/1 -> dotprod8/1
  dotprod8/1 -> Mux/8
  "IW{1,1}(9,:)'"/1 -> dotprod9/1
  dotprod9/1 -> Mux/9
  "IW{1,1}(10,:)'"/1 -> dotprod10/1
  dotprod10/1 -> Mux/10
  "IW{1,1}(11,:)'"/1 -> dotprod11/1
  dotprod11/1 -> Mux/11
  "IW{1,1}(12,:)'"/1 -> dotprod12/1
  dotprod12/1 -> Mux/12
  "IW{1,1}(13,:)'"/1 -> dotprod13/1
  dotprod13/1 -> Mux/13
  "IW{1,1}(14,:)'"/1 -> dotprod14/1
  dotprod14/1 -> Mux/14
  "IW{1,1}(15,:)'"/1 -> dotprod15/1
  dotprod15/1 -> Mux/15
  "IW{1,1}(16,:)'"/1 -> dotprod16/1
  dotprod16/1 -> Mux/16
  "IW{1,1}(17,:)'"/1 -> dotprod17/1
  dotprod17/1 -> Mux/17
  "IW{1,1}(18,:)'"/1 -> dotprod18/1
  dotprod18/1 -> Mux/18
  "IW{1,1}(19,:)'"/1 -> dotprod19/1
  dotprod19/1 -> Mux/19
  "IW{1,1}(20,:)'"/1 -> dotprod20/1
  dotprod20/1 -> Mux/20
  Mux/1 -> "iz{1,1}"/1

== system tutorial_switched_nets/NN_cex_1/Layer 2/Delays 1 ==
  "p{2}" : Inport  PortDimensions=20
      mask Display: e = 0.06;c1 = [120 230 180]/255;c2 = ([120 230 180]+0)/(256+128);c3 = ([120 230 180]+128)/(256+128);patch([0 1 1 0],[0 0 1 1],c1);patch([0 1 1 1-e 1-e 0+e],[0 0 1 1-e 0+e 0+e],c2);patch([0 0 1 1-e 0+e 0+e],[0 1 1 1-e 1-e 0+e],c3);plot([0 1 1 0 0],[0 0 1 1 0]);
  mux : Mux  Inputs=1
      mask Display: e = 0.06;c1 = [120 150 230]/255;c2 = ([120 150 230]+0)/383;c3 = ([120 150 230]+128)/383;patch([0 1 1 0],[0 0 1 1],c1);patch([0 1 1 1-e 1-e 0+e],[0 0 1 1-e 0+e 0+e],c2);patch([0 0 1 1-e 0+e 0+e],[0 1 1 1-e 1-e 0+e],c3);plot([0 1 1 0 0],[0 0 1 1 0]);disp('Mux')
  "pd{2,1}" : Outport
      mask Display: e = 0.06;c1 = [120 230 180]/255;c2 = ([120 230 180]+0)/(256+128);c3 = ([120 230 180]+128)/(256+128);patch([0 1 1 0],[0 0 1 1],c1);patch([0 1 1 1-e 1-e 0+e],[0 0 1 1-e 0+e 0+e],c2);patch([0 0 1 1-e 0+e 0+e],[0 1 1 1-e 1-e 0+e],c3);plot([0 1 1 0 0],[0 0 1 1 0]);
  wires:
  "p{2}"/1 -> mux/1
  mux/1 -> "pd{2,1}"/1
